simulink model "PitchControl"  (R2024b)
settings: Solver=VariableStepAuto  StartTime=0.0  StopTime=3  RelTol=1e-3
undefined symbols (not defined in the file or in its folder): Kd, Ki, Kp
libraries: slpidlib x1
settings Model: Creator=Arghya  LastModifiedBy=Arghya

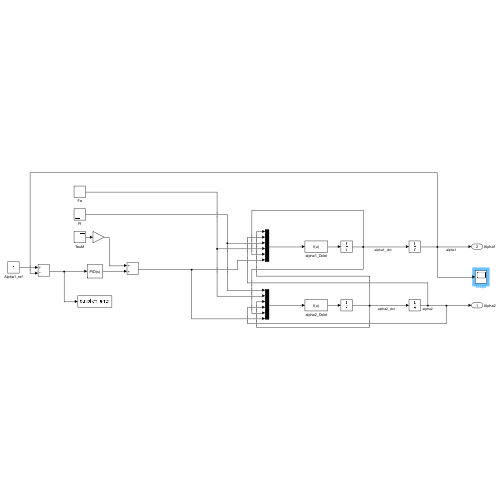
[thumbnail: Simulink's stored preview of the top-level diagram]
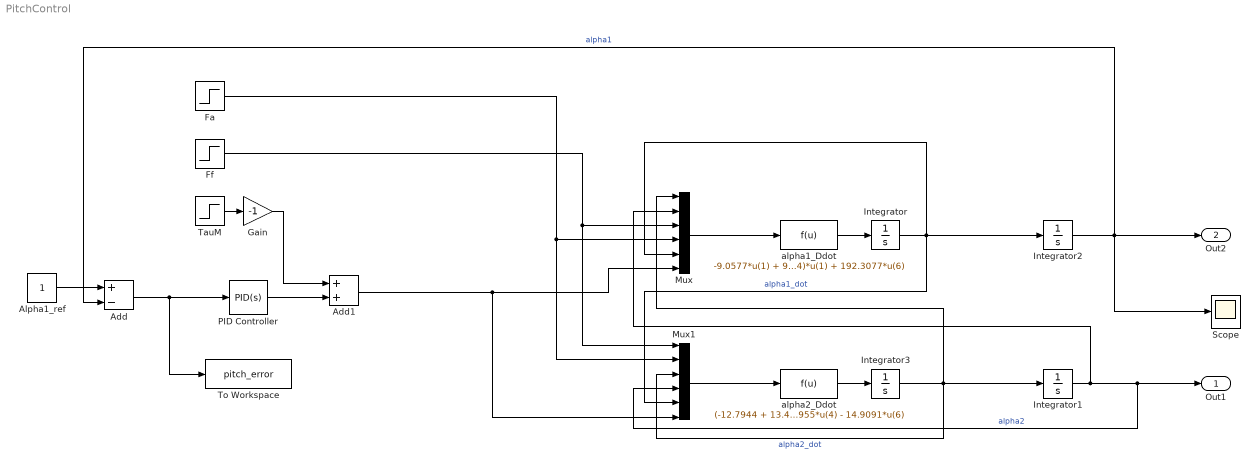
== system PitchControl ==
  Add : Sum  Inputs=+-
  Add1 : Sum
  Alpha1_ref : Constant
  Fa : Step  SampleTime=0.2
  Ff : Step  SampleTime=0.2
  Gain : Gain  Gain=-1
  Integrator : Integrator  UpperSaturationLimit=pi  LowerSaturationLimit=0  ContinuousStateAttributes="\"alpha1_dot\""
  Integrator1 : Integrator  ContinuousStateAttributes="\"alpha2\""
  Integrator2 : Integrator  ContinuousStateAttributes="\"alpha1\""
  Integrator3 : Integrator  UpperSaturationLimit=pi/2  LowerSaturationLimit=-pi/2  ContinuousStateAttributes="\"alpha2_dot\""
  Mux : Mux  Inputs=6
  Mux1 : Mux  Inputs=6
  PID Controller : slpidlib/PID Controller  Controller=PID  Form=Parallel  TimeDomain=Continuous-time  UseExternalTs=off  SampleTime=-1  IntegratorMethod=Forward Euler  FilterMethod=Forward Euler  ControllerParametersSource=internal  P=Kp  I=Ki  UseKiTs=off  D=Kd  UseExternalDerivativeSource=off  N=100  UseFilter=on  TunerSelectOption=Transfer Function Based (PID Tuner App)  InitialConditionSource=internal  InitialConditionForIntegrator=0  InitialConditionForFilter=0  DifferentiatorICPrevScaledInput=0  ExternalReset=none  TrackingMode=off  Kt=1  LimitOutput=off  SatLimitsSource=internal  UpperSaturationLimit=inf  LowerSaturationLimit=-inf  LinearizeAsGain=on  AntiWindupMode=none  Kb=1  LimitIntegrator=off  UpperIntegratorSaturationLimit=inf  LowerIntegratorSaturationLimit=-inf  POutMin=[]  POutMax=[]  IOutMin=[]  IOutMax=[]  DOutMin=[]  DOutMax=[]  NOutMin=[]  NOutMax=[]  SumOutMin=[]  SumOutMax=[]  SaturationOutMin=[]  SaturationOutMax=[]  PParamMin=[]  PParamMax=[]  IParamMin=[]  IParamMax=[]  DParamMin=[]  DParamMax=[]  NParamMin=[]  NParamMax=[]  KbParamMin=[]  KbParamMax=[]  KtParamMin=[]  KtParamMax=[]  KbOutMin=[]  KbOutMax=[]  KtOutMin=[]  KtOutMax=[]  IntegratorOutMin=[]  IntegratorOutMax=[]  FilterOutMin=[]  FilterOutMax=[]  SumI1OutMin=[]  SumI1OutMax=[]  SumI2OutMin=[]  SumI2OutMax=[]  SumI3OutMin=[]  SumI3OutMax=[]  SumI4OutMin=[]  SumI4OutMax=[]  SumDOutMin=[]  SumDOutMax=[]  DifferentiatorOutMin=[]  DifferentiatorOutMax=[]  FilterDiffOutCoefMin=[]  FilterDiffOutCoefMax=[]  ReciprocalOutMin=[]  ReciprocalOutMax=[]  SumDenOutMin=[]  SumDenOutMax=[]  SumNumOutMin=[]  SumNumOutMax=[]  DivideOutMin=[]  DivideOutMax=[]  UdiffTsProdOutMin=[]  UdiffTsProdOutMax=[]  NTsProdOutMin=[]  NTsProdOutMax=[]  UintegralTsProdOutMin=[]  UintegralTsProdOutMax=[]  UngainTsProdOutMin=[]  UngainTsProdOutMax=[]  ClampingZeroOutDataTypeStr=Inherit: Inherit via back propagation  ClampingZeroOutMin=[]  ClampingZeroOutMax=[]  FilterDenConstantOutDataTypeStr=Inherit: Inherit via back propagation  FilterDenConstantOutMin=[]  FilterDenConstantOutMax=[]  PCopyOutDataTypeStr=Inherit: Inherit via back propagation  PCopyOutMin=[]  PCopyOutMax=[]  NCopyOutDataTypeStr=Inherit: Inherit via back propagation  NCopyOutMin=[]  NCopyOutMax=[]  IntegratorContinuousStateAttributes=''  IntegratorStateMustResolveToSignalObject=off  IntegratorRTWStateStorageClass=Auto  FilterContinuousStateAttributes=''  FilterStateMustResolveToSignalObject=off  FilterRTWStateStorageClass=Auto  ParallelPVariant=InternalParameters  IdealPVariant=Disabled  IVariant=InternalParameters  DVariant=InternalParameters  IntegratorVariant=Continuous  SatVariant=Disabled  AWVariant=Passthrough  PCopyVariant=Disabled  TRVariant=Disabled  FdbkBlocksVariant=Forward  IdealPFdbkVariant=Disabled  SatFdbkVariant=Disabled  DerivativeFilterVariant=ContFilter  NVariant=InternalParameters  NCopyVariant=Disabled  FilterICVariant=InternalICsFilter  IntegratorICVariant=InternalICs  ExternalResetVariant=Disabled  TRSumVariant=Passthrough  SumFdbkVariant=Disabled  SumVariant=Sum_PID  TsampFilterVariant=InternalTs  TsampNgainVariant=Passthrough  TsampIntegralVariant=Disabled_SignalSpec  ExternalSaturationOutDataTypeStr=Inherit: Same as second input  DerivativeSourceVariant=ErrorSignal  PreIntVariant=InternalPreInt
  Scope : Scope
  TauM : Step  SampleTime=0.2
  To Workspace : ToWorkspace  VariableName=pitch_error  SampleTime=-1
  alpha1_Ddot : Fcn  Expr=-9.0577*u(1) + 9.0577*u(2)*u(1)*u(1) - 192.3077*(u(3)+u(4))*u(5) + 192.3077*u(4)*u(1) + 192.3077*u(6)
  alpha2_Ddot : Fcn  Expr=(-12.7944 + 13.4268*u(1) + 11.944*u(2))*u(3) - 0.6324*u(4)*u(3)*u(3) + 1.4824*u(5) + 12.1955*u(4) - 14.9091*u(6)
  Out1 : Outport  SignalName=Alpha2
  Out2 : Outport  Port=2  SignalName=Alpha1
  wires:
  Integrator/1 -> Mux1/5, Mux/5, Integrator2/1  "alpha1_dot"
  alpha1_Ddot/1 -> Integrator/1
  Integrator3/1 -> Mux/1, Mux1/3, Integrator1/1  "alpha2_dot"
  alpha2_Ddot/1 -> Integrator3/1
  Integrator2/1 -> Scope/1, Add/2, Out2/1  "alpha1"
  Integrator1/1 -> Mux/2, Mux1/4, Out1/1  "alpha2"
  Ff/1 -> Mux1/1, Mux/3
  Fa/1 -> Mux1/2, Mux/4
  Mux/1 -> alpha1_Ddot/1
  Mux1/1 -> alpha2_Ddot/1
  TauM/1 -> Gain/1
  Gain/1 -> Add1/1
  Alpha1_ref/1 -> Add/1
  Add/1 -> To Workspace/1, PID Controller/1
  PID Controller/1 -> Add1/2
  Add1/1 -> Mux1/6, Mux/6
